simulink library "hcu_lib"  (Simulink 8.6)
settings: Solver=ode45  SolverMode=SingleTasking  StartTime=0.0  StopTime=10.0  RelTol=1e-3
PreLoadFcn:
  | if exist('tl_preloadfcn','file'), tl_preloadfcn(gcs,100); end
PostLoadFcn:
  | if exist('tl_postloadfcn','file'), tl_postloadfcn(gcs,100); end
undefined symbols (not defined in the file or in its folder): C_TICK_TIME_S, DEG2RAD, EPSILON, FALSE, RAD2DEG, TRUE
undefined symbols (not defined in the file): UNDEFINED_VALUE
libraries: hcu_lib x19, simulink x4
(part 1 of 3)
settings Model: TLRevision=100  Creator=gpf  LastModifiedBy=14069  ExtModeAutoUpdateStatusClock=off

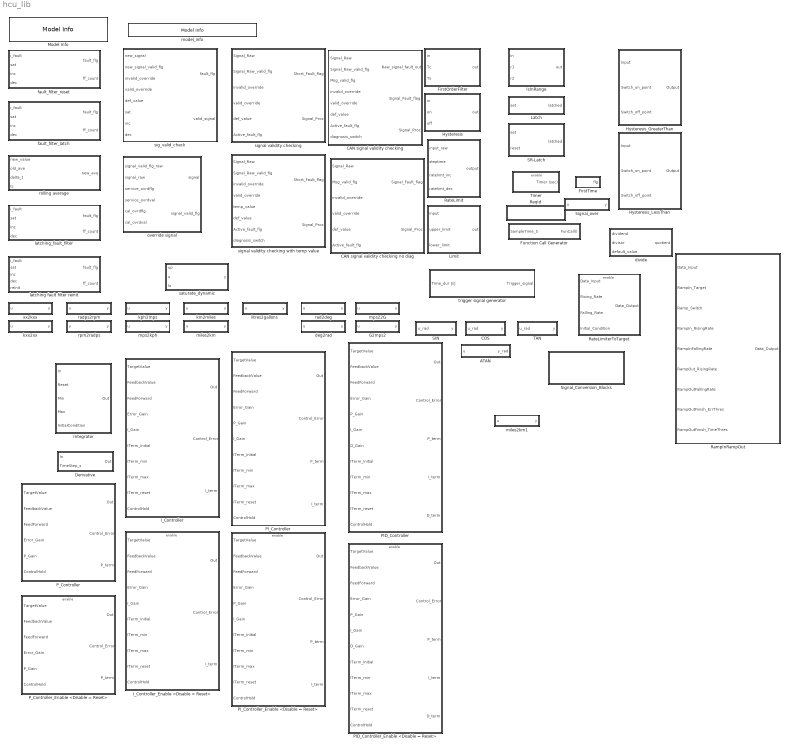
== system hcu_lib ==
  ATAN : Subsystem  TreatAsAtomicUnit=on  RTWFcnName=atan_lib  RTWFileName=HCU_LIB  mask(Inverse Trigonometric Function (ArcTangent)){}
      mask help:
      | Calculate aTan of the Input Signal.
      | The unit of output signal is rad.
      | If input signal is greater than 1000, it would be regard as PI rad.
      | If input signal is less than -1000, it would be regarded as -PI rad.
      | The output is bounded between -PI rad to PI rad.
      settings: RTWFcnNameOpts=User specified  RTWFileNameOpts=User specified
      mask Display:
      | disp('ATAN(X)' , 'texmode', 'on');
      | port_label('output',1,'Y_rad');
      | port_label('input',1,'X')
  CAN signal validity checking : Subsystem  TreatAsAtomicUnit=on  RTWFcnName=can_sig_valid_check  RTWFileName=HCU_LIB
      settings: RTWFcnNameOpts=User specified  RTWFileNameOpts=User specified
  CAN signal validity checking no diag : Subsystem  TreatAsAtomicUnit=on  RTWFcnName=can_sig_valid_check_no_diag  RTWFileName=HCU_LIB
      settings: RTWFcnNameOpts=User specified  RTWFileNameOpts=User specified
  COS : Subsystem  TreatAsAtomicUnit=on  RTWFcnName=cos_lib  RTWFileName=HCU_LIB  mask(Trigonometric Function (Cosine)){}
      mask help:
      | Calculate Cos of the Input Signal.
      | The unit of input signal is rad.
      settings: RTWFcnNameOpts=User specified  RTWFileNameOpts=User specified
      mask Display:
      | disp('       COS(X)' , 'texmode', 'on');
      | port_label('output',1,'Y');
      | port_label('input',1,'X_rad')
  Derivative : Subsystem  TreatAsAtomicUnit=on  RTWFcnName=derivative_lib  RTWFileName=HCU_LIB
      settings: RTWFcnNameOpts=User specified  RTWFileNameOpts=User specified
      mask Display: disp('Derivative')
  FirstOrderFilter : Subsystem  TreatAsAtomicUnit=on  RTWFcnName=firstorderfilter_lib  RTWFileName=HCU_LIB
      settings: RTWFcnNameOpts=User specified  RTWFileNameOpts=User specified
  FirstTime : Subsystem  TreatAsAtomicUnit=on  RTWFcnName=firsttime_lib  RTWFileName=HCU_LIB  mask(First Time True){}
      mask help: The output is TRUE if first time executing the block.
      settings: RTWFcnNameOpts=User specified  RTWFileNameOpts=User specified
  Function Call Generator : Stateflow chart  TreatAsAtomicUnit=on
  G2mps2 : Subsystem  TreatAsAtomicUnit=on  RTWFcnName=G2mps2_lib  RTWFileName=HCU_LIB  mask(Conversion){}
      mask help: Convert G to Meter per second^2.
      settings: RTWFcnNameOpts=User specified  RTWFileNameOpts=User specified
      mask Display: disp('G \rightarrow m/s2', 'texmode', 'on')
  Hysteresis : Subsystem  TreatAsAtomicUnit=on  RTWFcnName=hysteresis_lib  RTWFileName=HCU_LIB
      settings: RTWFcnNameOpts=User specified  RTWFileNameOpts=User specified
  Hysteresis_GreaterThan : Subsystem  TreatAsAtomicUnit=on  RTWFcnName=hysteresisgreaterthan_lib  RTWFileName=HCU_LIB
      settings: RTWFcnNameOpts=User specified  RTWFileNameOpts=User specified
  Hysteresis_LessThan : Subsystem  TreatAsAtomicUnit=on  RTWFcnName=hysteresislessthan_lib  RTWFileName=HCU_LIB
      settings: RTWFcnNameOpts=User specified  RTWFileNameOpts=User specified
  I_Controller : Subsystem  TreatAsAtomicUnit=on  RTWFcnName=icontroller_lib  RTWFileName=HCU_LIB
      settings: RTWFcnNameOpts=User specified  RTWFileNameOpts=User specified
      mask Display: disp('I Controller')
  I_Controller_Enable <Disable = Reset> : Subsystem  TreatAsAtomicUnit=on  RTWFcnName=icontrollerenable_lib  RTWFileName=HCU_LIB
      settings: RTWFcnNameOpts=User specified  RTWFileNameOpts=User specified
      mask Display: disp('I Controller\nwith Enable')
  Integrator : Subsystem  TreatAsAtomicUnit=on  RTWFcnName=integrator_lib  RTWFileName=HCU_LIB
      settings: RTWFcnNameOpts=User specified  RTWFileNameOpts=User specified
      mask Display: disp('Integrator')
  IsInRange : Subsystem  TreatAsAtomicUnit=on  RTWFcnName=isinrange_lib  RTWFileName=HCU_LIB
      settings: RTWFcnNameOpts=User specified  RTWFileNameOpts=User specified
  Latch : Subsystem  TreatAsAtomicUnit=on  RTWFcnName=latch_lib  RTWFileName=HCU_LIB
      settings: RTWFcnNameOpts=User specified  RTWFileNameOpts=User specified
  Limit : Subsystem  TreatAsAtomicUnit=on  RTWFcnName=limit_lib  RTWFileName=HCU_LIB
      settings: RTWFcnNameOpts=User specified  RTWFileNameOpts=User specified
  Model Info : simulink/Model-Wide Utilities/Model Info  BlockCM=None  Frame=on  DisplayStringWithTags=|  HorizontalTextAlignment=Left  LeftAlignmentValue=0.02  SourceBlockDiagram=hcu_lib  TagMaxNumber=20
      | Model Version        : %<ModelVersion>
      | Creator                   : %<Creator>
      | Last Modified by    : %<LastModifiedBy>
  PID_Controller : Subsystem  TreatAsAtomicUnit=on  RTWFcnName=pidcontroller_lib  RTWFileName=HCU_LIB
      settings: RTWFcnNameOpts=User specified  RTWFileNameOpts=User specified
      mask Display: disp('PID Controller')
  PID_Controller_Enable <Disable = Reset> : Subsystem  TreatAsAtomicUnit=on  RTWFcnName=pidcontrollerenable_lib  RTWFileName=HCU_LIB
      settings: RTWFcnNameOpts=User specified  RTWFileNameOpts=User specified
      mask Display: disp('PID Controller\nwith Enable')
  PI_Controller : Subsystem  TreatAsAtomicUnit=on  RTWFcnName=picontroller_lib  RTWFileName=HCU_LIB
      settings: RTWFcnNameOpts=User specified  RTWFileNameOpts=User specified
      mask Display: disp('PI Controller')
  PI_Controller_Enable <Disable = Reset> : Subsystem  TreatAsAtomicUnit=on  RTWFcnName=picontrollerenable_lib  RTWFileName=HCU_LIB
      settings: RTWFcnNameOpts=User specified  RTWFileNameOpts=User specified
      mask Display: disp('PI Controller\nwith Enable')
  P_Controller : Subsystem  TreatAsAtomicUnit=on  RTWFcnName=pcontroller_lib  RTWFileName=HCU_LIB
      settings: RTWFcnNameOpts=User specified  RTWFileNameOpts=User specified
      mask Display: disp('P Controller')
  P_Controller_Enable <Disable = Reset> : Subsystem  TreatAsAtomicUnit=on  RTWFcnName=pcontrollerenable_lib  RTWFileName=HCU_LIB
      settings: RTWFcnNameOpts=User specified  RTWFileNameOpts=User specified
      mask Display: disp('P Controller\nwith Enable')
  RampInRampOut : Subsystem  TreatAsAtomicUnit=on  RTWFcnName=rampinrampout_lib  RTWFileName=HCU_LIB
      settings: RTWFcnNameOpts=User specified  RTWFileNameOpts=User specified
  RateLimit : Subsystem  TreatAsAtomicUnit=on  RTWFcnName=ratelimit_lib  RTWFileName=HCU_LIB
      settings: RTWFcnNameOpts=User specified  RTWFileNameOpts=User specified
  RateLimiterToTarget : Subsystem  RTWFcnName=ratelimitertotarget_lib  RTWFileName=HCU_LIB
      settings: RTWFcnNameOpts=User specified  RTWFileNameOpts=User specified
  ReqId : Subsystem  mask(ReqId){req_str=HCU_000}
      mask prompts: req_str "Requirement:"
      mask help: Requirement Id
      mask Display: disp(sprintf('ReqId: %s',req_str));
  SIN : Subsystem  TreatAsAtomicUnit=on  RTWFcnName=sin_lib  RTWFileName=HCU_LIB  mask(Trigonometric Function (Sine)){}
      mask help:
      | Calculate Sin of the Input Signal.
      | The unit of input signal is rad.
      settings: RTWFcnNameOpts=User specified  RTWFileNameOpts=User specified
      mask Display:
      | disp('      SIN(X)' , 'texmode', 'on');
      | port_label('output',1,'Y');
      | port_label('input',1,'X_rad')
  SR-Latch : Subsystem  TreatAsAtomicUnit=on  RTWFcnName=srlatch_lib  RTWFileName=HCU_LIB
      settings: RTWFcnNameOpts=User specified  RTWFileNameOpts=User specified
  Signal_Conversion_Blocks : Subsystem
  Signal_over : Subsystem  mask(Override){parent_name=Signal, cal=0}
      mask prompts: parent_name "Name"; cal "Set Value"
      mask help: Override signal
      mask Callback parent_name: set_param(gcb, 'name', [get_param(gcb, 'parent_name') '_over']);
      mask Display: disp('Override');
  TAN : Subsystem  TreatAsAtomicUnit=on  RTWFcnName=tan_lib  RTWFileName=HCU_LIB  mask(Trigonometric Function (Tangent)){}
      mask help:
      | Calculate Tan of the Input Signal.
      | The unit of input signal is rad.
      settings: RTWFcnNameOpts=User specified  RTWFileNameOpts=User specified
      mask Display:
      | disp('      TAN(X)' , 'texmode', 'on');
      | port_label('output',1,'Y');
      | port_label('input',1,'X_rad')
  Timer : Subsystem  TreatAsAtomicUnit=on  RTWFcnName=timer_lib  RTWFileName=HCU_LIB
      settings: RTWFcnNameOpts=User specified  RTWFileNameOpts=User specified
  deg2rad : Subsystem  TreatAsAtomicUnit=on  RTWFcnName=deg2rad_lib  RTWFileName=HCU_LIB  mask(Conversion){}
      mask help: Convert degs to rads.
      settings: RTWFcnNameOpts=User specified  RTWFileNameOpts=User specified
      mask Display: disp('deg \rightarrow rad', 'texmode', 'on')
  divide : Subsystem  TreatAsAtomicUnit=on  RTWFcnName=divide_lib  RTWFileName=HCU_LIB  mask(divide){}
      mask help: Performs a division operation. If the divisor is found to be between -0.00001 and +0.00001 then a failsafe value is passed to the output.
      settings: RTWFcnNameOpts=User specified  RTWFileNameOpts=User specified
      mask Display: disp('Divide');
  fault_filter_latch : Subsystem  TreatAsAtomicUnit=on  RTWFcnName=ff_latch  RTWFileName=HCU_LIB
      settings: RTWFcnNameOpts=Use subsystem name  RTWFileNameOpts=User specified
  fault_filter_reset : Subsystem  TreatAsAtomicUnit=on  RTWFcnName=ff_reset  RTWFileName=HCU_LIB
      settings: RTWFcnNameOpts=User specified  RTWFileNameOpts=User specified
  km2miles : Subsystem  TreatAsAtomicUnit=on  RTWFcnName=km2miles_lib  RTWFileName=HCU_LIB  mask(Conversion){}
      mask help: Convert kilometers to miles.
      settings: RTWFcnNameOpts=User specified  RTWFileNameOpts=User specified
      mask Display: disp('km \rightarrow mile', 'texmode', 'on')
  kph2mps : Subsystem  TreatAsAtomicUnit=on  RTWFcnName=kph2mps_lib  RTWFileName=HCU_LIB  mask(Conversion){}
      mask help: Convert Kilometers per hour to Meters per second
      settings: RTWFcnNameOpts=User specified  RTWFileNameOpts=User specified
      mask Display: disp('km/h \rightarrow m/s', 'texmode', 'on')
  kxx2xx : Subsystem  TreatAsAtomicUnit=on  RTWFcnName=kxx2xx_lib  RTWFileName=HCU_LIB  mask(Conversion){}
      mask help: Multiply by 1000.
      settings: RTWFcnNameOpts=User specified  RTWFileNameOpts=User specified
      mask Display: disp('kiloxx \rightarrow xx', 'texmode', 'on')
  latching fault filter reinit : Subsystem  TreatAsAtomicUnit=on  RTWFcnName=ff_latching  RTWFileName=HCU_LIB  mask(Latching Fault Filter){}
      mask help: Fault filter block - Latches the fault output flag to TRUE if the input flag is repeatedly set True.
      settings: RTWFcnNameOpts=User specified  RTWFileNameOpts=User specified
      mask Display: disp('Latching\nFault Filter')
  latching_fault_filter : Subsystem  TreatAsAtomicUnit=on  RTWFcnName=ff_latching  RTWFileName=HCU_LIB  mask(Latching Fault Filter){}
      mask help: Fault filter block - Latches the fault output flag to TRUE if the input flag is repeatedly set True.
      settings: RTWFcnNameOpts=User specified  RTWFileNameOpts=User specified
      mask Display: disp('Latching\nFault Filter')
  litres2gallons : Subsystem  TreatAsAtomicUnit=on  RTWFcnName=liters2gallons_lib  RTWFileName=HCU_LIB  mask(Conversion){UK=off}
      mask prompts: UK "UK Gallon"
      mask help: Convert litres to gallons.
      settings: RTWFcnNameOpts=User specified  RTWFileNameOpts=User specified
      mask Display: disp('litre \rightarrow gallon', 'texmode', 'on')
  miles2km : Subsystem  TreatAsAtomicUnit=on  RTWFcnName=miles2km_lib  RTWFileName=HCU_LIB  mask(Conversion){}
      mask help: Convert kilometers to miles.
      settings: RTWFcnNameOpts=User specified  RTWFileNameOpts=User specified
      mask Display: disp('mile \rightarrow km', 'texmode', 'on')
  miles2km1 : Subsystem  mask(Conversion){}
      mask help: Convert degs to rads.
      mask Display: disp('deg \rightarrow rad', 'texmode', 'on')
  model_info : simulink/Model-Wide Utilities/Model Info  BlockCM=None  Frame=on  DisplayStringWithTags=$Id: hcu_lib.mdl 2 2019-09-19 09:28:50Z JuneXmas $  HorizontalTextAlignment=Center  LeftAlignmentValue=0.5  SourceBlockDiagram=hcu_lib  TagMaxNumber=20
  mps22G : Subsystem  TreatAsAtomicUnit=on  RTWFcnName=mps22G_lib  RTWFileName=HCU_LIB  mask(Conversion){}
      mask help: Convert Meter per second^2 to G.
      settings: RTWFcnNameOpts=User specified  RTWFileNameOpts=User specified
      mask Display: disp('m/s2 \rightarrow G', 'texmode', 'on')
  mps2kph : Subsystem  TreatAsAtomicUnit=on  RTWFcnName=mps2kph_lib  RTWFileName=HCU_LIB  mask(Conversion){}
      mask help: Convert Meters per second to Kilometers per hour
      settings: RTWFcnNameOpts=User specified  RTWFileNameOpts=User specified
      mask Display: disp('m/s \rightarrow km/h', 'texmode', 'on')
  override signal : Subsystem  RTWFcnName=srvc_ovrd  RTWFileName=HCU_LIB
      settings: RTWSystemCode=Inline  RTWFcnNameOpts=User specified  RTWFileNameOpts=User specified
  rad2deg : Subsystem  TreatAsAtomicUnit=on  RTWFcnName=rad2deg_lib  RTWFileName=HCU_LIB  mask(Conversion){}
      mask help: Convert rads to degs.
      settings: RTWFcnNameOpts=User specified  RTWFileNameOpts=User specified
      mask Display: disp('rad \rightarrow deg', 'texmode', 'on')
  radps2rpm : Subsystem  TreatAsAtomicUnit=on  RTWFcnName=radps2rpm_lib  RTWFileName=HCU_LIB
      mask help: Converst radians per second to revolutions per minute.
      settings: RTWFcnNameOpts=User specified  RTWFileNameOpts=User specified
      mask Display: disp('rad/s \rightarrow rpm', 'texmode', 'on')
  rolling average : Subsystem  TreatAsAtomicUnit=on  RTWFcnName=rolav_tc  RTWFileName=HCU_LIB  mask(Rolling Average){}
      mask help:
      | Rolling Average - Time Constant.  This filter block is the first order approximation using a time constant.  Inputs include the time constant (entered through this dialogue), old_ave which is the previous average value, new_value which is the new filter to filter toward.
      |
      | The sample_interval which is elapsed time over which to perform the filter equation is computed internally - THIS BLOCK MUST BE CALLED EACH PASS to work as expected.
      settings: RTWFcnNameOpts=User specified  RTWFileNameOpts=User specified
      mask Display: disp('Rolling Average - TC')
  rpm2radps : Subsystem  TreatAsAtomicUnit=on  RTWFcnName=rpm2radps_lib  RTWFileName=HCU_LIB
      mask help: Converts revolutions per minute to radians per second.
      settings: RTWFcnNameOpts=User specified  RTWFileNameOpts=User specified
      mask Display: disp('rpm \rightarrow rad/s', 'texmode', 'on')
  saturate_dynamic : Subsystem  TreatAsAtomicUnit=on  RTWFcnName=saturatedynamic_lib  RTWFileName=HCU_LIB  mask(saturate_dynamic){}
      mask help: Limit input signal in dynamic upper and lower limits
      settings: RTWFcnNameOpts=User specified  RTWFileNameOpts=User specified
      mask Display: disp('Saturate_Dynamic');
  sig_valid_check : Subsystem  TreatAsAtomicUnit=on  RTWFcnName=sig_valid_check  RTWFileName=HCU_LIB
      settings: RTWFcnNameOpts=User specified  RTWFileNameOpts=User specified
  signal validity checking : Subsystem  TreatAsAtomicUnit=on  RTWFcnName=sig_valid_check  RTWFileName=HCU_LIB
      settings: RTWFcnNameOpts=User specified  RTWFileNameOpts=User specified
  signal validity checking with temp value : Subsystem  TreatAsAtomicUnit=on  RTWFcnName=sig_valid_check_with_temp_value  RTWFileName=HCU_LIB
      settings: RTWFcnNameOpts=User specified  RTWFileNameOpts=User specified
  trigger signal generator : Subsystem  TreatAsAtomicUnit=on
  xx2kxx : Subsystem  TreatAsAtomicUnit=on  RTWFcnName=xx2kxx_lib  RTWFileName=HCU_LIB  mask(Conversion){}
      mask help: Divides by 1000.
      settings: RTWFcnNameOpts=User specified  RTWFileNameOpts=User specified
      mask Display: disp('xx \rightarrow kiloxx', 'texmode', 'on')

== system hcu_lib/ATAN ==
  u : Inport
  ATAN_Function_NEG : Lookup_n-D  NumberOfTableDimensions=1  BreakpointsForDimension1="[-1000\t-11.4300523\t-5.67128182\t-3.732050808\t-1.732050808\t-1\t-0.577350269\t-0.267949192\t-0.176326981\t-0.087488664\t0]"  Table="[-90\t-85\t-80\t-75\t-60\t-45\t-30\t-15\t-10\t-5\t0]"  ExtrapMethod=Clip  UseLastTableValue=on  InternalRulePriority=Speed  RndMeth=Simplest  InputSameDT=on
  ATAN_Function_POS : Lookup_n-D  NumberOfTableDimensions=1  BreakpointsForDimension1="[0\t0.087488664\t0.176326981\t0.267949192\t0.577350269\t1\t1.732050808\t3.732050808\t5.67128182\t11.4300523\t1000]"  Table="[0\t5\t10\t15\t30\t45\t60\t75\t80\t85\t90]"  ExtrapMethod=Clip  UseLastTableValue=on  InternalRulePriority=Speed  RndMeth=Simplest  InputSameDT=on
  Compare To Zero : simulink/Logic and Bit Operations/Compare To Zero  relop=>=  OutDataTypeStr=boolean
  Saturation : Saturate  UpperLimit=1000  LowerLimit=0
  Saturation1 : Saturate  UpperLimit=0  LowerLimit=-1000
  Switch : Switch  Criteria=u2 ~= 0
  deg2rad : hcu_lib/deg2rad
  y_rad : Outport
  wires:
  ATAN_Function_POS/1 -> Switch/1
  Saturation/1 -> ATAN_Function_POS/1
  Saturation1/1 -> ATAN_Function_NEG/1
  u/1 -> Saturation/1, Compare To Zero/1, Saturation1/1
  ATAN_Function_NEG/1 -> Switch/3
  Compare To Zero/1 -> Switch/2
  Switch/1 -> deg2rad/1
  deg2rad/1 -> y_rad/1

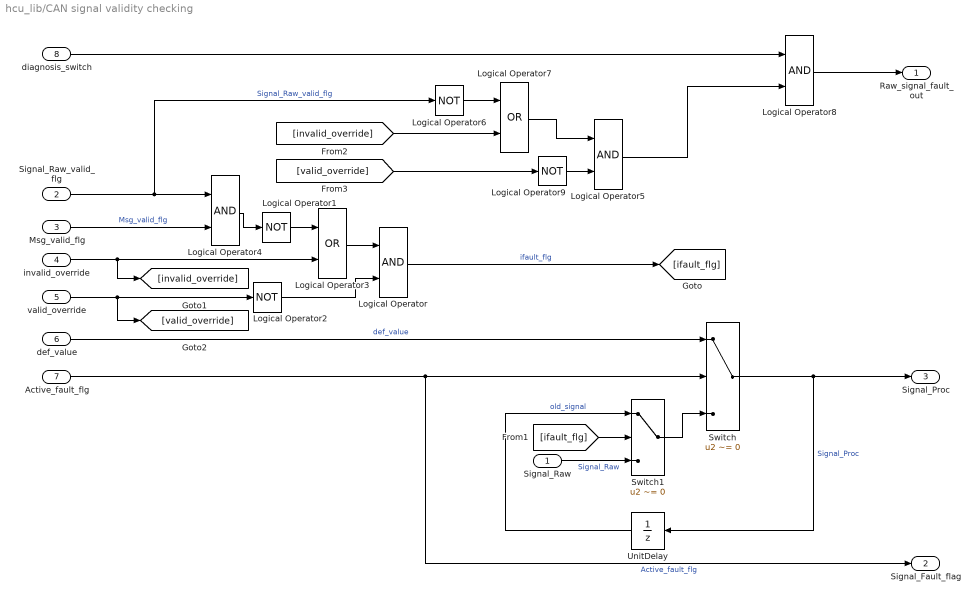
== system hcu_lib/CAN signal validity checking ==
  Signal_Raw : Inport
  Signal_Raw_valid_flg : Inport  Port=2
  Msg_valid_flg : Inport  Port=3
  invalid_override : Inport  Port=4
  valid_override : Inport  Port=5
  def_value : Inport  Port=6
  Active_fault_flg : Inport  Port=7
  diagnosis_switch : Inport  Port=8
  Logical Operator{,4..5,8} (4 alike) : Logic  Tag=struct('inputs','2','comment',struct('text','','placement',1),'logdata',struct('maxnumvals',inf,'plotchannels',[],'stepsize',0,'downsampling',1,'loggingmode',3,'channels',1),'operator','OR','output',struct('class','default','type','Bool8','description','','address','','unit','','name','$S_$B'),'date',731430.467498704)
  Logical Operator{1..2,6,9} (4 alike) : Logic  Tag=struct('inputs','1','comment',struct('text','','placement',1),'logdata',struct('maxnumvals',inf,'plotchannels',[],'stepsize',0,'downsampling',1,'loggingmode',3,'channels',1),'operator','NOT','output',struct('class','default','type','Bool8','description','','address','','unit','','name','$S_$B'),'date',731430.46749816)  Operator=NOT  Inputs=1
  Logical Operator3 : Logic  Tag=struct('inputs','2','comment',struct('text','','placement',1),'logdata',struct('maxnumvals',inf,'plotchannels',[],'stepsize',0,'downsampling',1,'loggingmode',3,'channels',1),'operator','OR','output',struct('class','default','type','Bool8','description','','address','','unit','','name','$S_$B'),'date',731430.467498704)  Operator=OR
  Logical Operator7 : Logic  Tag=struct('inputs','2','comment',struct('text','','placement',1),'logdata',struct('maxnumvals',inf,'plotchannels',[],'stepsize',0,'downsampling',1,'loggingmode',3,'channels',1),'operator','OR','output',struct('class','default','type','Bool8','description','','address','','unit','','name','$S_$B'),'date',731430.467498704)  Operator=OR
  Switch : Switch  Criteria=u2 ~= 0
  Switch1 : Switch  Criteria=u2 ~= 0
  UnitDelay : UnitDelay  Tag=struct('comment',struct('text','','placement',1),'logdata',struct('maxnumvals',inf,'plotchannels',[],'stepsize',0,'downsampling',1,'loggingmode',3,'channels',1),'output',struct('width',1,'name','$S_$B','unit','','type','Int32Bin15','offset',0,'max',32767,'min',-32768,'freeze',1,'lsb',2^-16,'arb',0,'class','default','address','','description','','autoscalingmode',1,'lowerheadroom',1,'upperheadroom',1,'headroomunit','bit','checkmin',0,'checkmax',0,'show',0,'initial','0'),'state',0,'dt','-1','date',731401.644401968)  SampleTime=-1
  Raw_signal_fault_out : Outport
  Signal_Fault_flag : Outport  Port=2
  Signal_Proc : Outport  Port=3
  wires:
  Logical Operator6/1 -> Logical Operator7/1
  Logical Operator9/1 -> Logical Operator5/2
  diagnosis_switch/1 -> Logical Operator8/1
  Logical Operator8/1 -> Raw_signal_fault_out/1
  Logical Operator5/1 -> Logical Operator8/2
  Logical Operator7/1 -> Logical Operator5/1
  [invalid_override] -> Logical Operator7/2
  [valid_override] -> Logical Operator9/1
  Logical Operator4/1 -> Logical Operator1/1
  Msg_valid_flg/1 -> Logical Operator4/2  "Msg_valid_flg"
  Switch/1 -> Signal_Proc/1, UnitDelay/1  "Signal_Proc"
  def_value/1 -> Switch/1  "def_value"
  Logical Operator1/1 -> Logical Operator3/1
  Signal_Raw_valid_flg/1 -> Logical Operator6/1, Logical Operator4/1  "Signal_Raw_valid_flg"
  invalid_override/1 -> [invalid_override], Logical Operator3/2
  Active_fault_flg/1 -> Signal_Fault_flag/1, Switch/2  "Active_fault_flg"
  UnitDelay/1 -> Switch1/1  "old_signal"
  Switch1/1 -> Switch/3
  Signal_Raw/1 -> Switch1/3  "Signal_Raw"
  Logical Operator/1 -> [ifault_flg]  "ifault_flg"
  [ifault_flg] -> Switch1/2
  valid_override/1 -> [valid_override], Logical Operator2/1
  Logical Operator3/1 -> Logical Operator/1
  Logical Operator2/1 -> Logical Operator/2

== system hcu_lib/CAN signal validity checking no diag ==
  Signal_Raw : Inport
  Msg_valid_flg : Inport  Port=2
  invalid_override : Inport  Port=3
  valid_override : Inport  Port=4
  def_value : Inport  Port=5
  Active_fault_flg : Inport  Port=6
  Logical Operator : Logic  Tag=struct('inputs','2','comment',struct('text','','placement',1),'logdata',struct('maxnumvals',inf,'plotchannels',[],'stepsize',0,'downsampling',1,'loggingmode',3,'channels',1),'operator','OR','output',struct('class','default','type','Bool8','description','','address','','unit','','name','$S_$B'),'date',731430.467498704)
  Logical Operator1 : Logic  Tag=struct('inputs','1','comment',struct('text','','placement',1),'logdata',struct('maxnumvals',inf,'plotchannels',[],'stepsize',0,'downsampling',1,'loggingmode',3,'channels',1),'operator','NOT','output',struct('class','default','type','Bool8','description','','address','','unit','','name','$S_$B'),'date',731430.46749816)  Operator=NOT  Inputs=1
  Logical Operator2 : Logic  Tag=struct('inputs','1','comment',struct('text','','placement',1),'logdata',struct('maxnumvals',inf,'plotchannels',[],'stepsize',0,'downsampling',1,'loggingmode',3,'channels',1),'operator','NOT','output',struct('class','default','type','Bool8','description','','address','','unit','','name','$S_$B'),'date',731430.46749816)  Operator=NOT  Inputs=1
  Logical Operator3 : Logic  Tag=struct('inputs','2','comment',struct('text','','placement',1),'logdata',struct('maxnumvals',inf,'plotchannels',[],'stepsize',0,'downsampling',1,'loggingmode',3,'channels',1),'operator','OR','output',struct('class','default','type','Bool8','description','','address','','unit','','name','$S_$B'),'date',731430.467498704)  Operator=OR
  Switch : Switch  Criteria=u2 ~= 0
  Switch1 : Switch  Criteria=u2 ~= 0
  UnitDelay : UnitDelay  Tag=struct('comment',struct('text','','placement',1),'logdata',struct('maxnumvals',inf,'plotchannels',[],'stepsize',0,'downsampling',1,'loggingmode',3,'channels',1),'output',struct('width',1,'name','$S_$B','unit','','type','Int32Bin15','offset',0,'max',32767,'min',-32768,'freeze',1,'lsb',2^-16,'arb',0,'class','default','address','','description','','autoscalingmode',1,'lowerheadroom',1,'upperheadroom',1,'headroomunit','bit','checkmin',0,'checkmax',0,'show',0,'initial','0'),'state',0,'dt','-1','date',731401.644401968)  SampleTime=-1
  Signal_Fault_flag : Outport
  Signal_Proc : Outport  Port=2
  wires:
  Msg_valid_flg/1 -> Logical Operator1/1  "Msg_valid_flg"
  Switch/1 -> Signal_Proc/1, UnitDelay/1  "Signal_Proc"
  def_value/1 -> Switch/1  "def_value"
  Logical Operator1/1 -> Logical Operator3/1
  invalid_override/1 -> Logical Operator3/2
  Active_fault_flg/1 -> Signal_Fault_flag/1, Switch/2  "Active_fault_flg"
  UnitDelay/1 -> Switch1/1  "old_signal"
  Switch1/1 -> Switch/3
  Signal_Raw/1 -> Switch1/3  "Signal_Raw"
  Logical Operator/1 -> [ifault_flg]  "ifault_flg"
  [ifault_flg] -> Switch1/2
  valid_override/1 -> Logical Operator2/1
  Logical Operator3/1 -> Logical Operator/1
  Logical Operator2/1 -> Logical Operator/2

== system hcu_lib/COS ==
  u_rad : Inport
  COS_Function : Lookup_n-D  NumberOfTableDimensions=1  BreakpointsForDimension1="[0\t5\t10\t15\t30\t45\t60\t75\t80\t85\t90\t95\t100\t105\t120\t135\t150\t165\t170\t175\t180\t185\t190\t195\t210\t225\t240\t255\t260\t265\t270\t275\t280\t285\t300\t315\t330\t345\t350\t355\t360]"  Table="[1\t0.996194698\t0.984807753\t0.965925826\t0.866025404\t0.707106781\t0.5\t0.258819045\t0.173648178\t0.087155743\t0\t-0.087155743\t-0.173648178\t-0.258819045\t-0.5\t-0.707106781\t-0.866025404\t-0.965925826\t-0.984807753\t-0.996194698\t-1\t-0.996194698\t-0.984807753\t-0.965925826\t-0.866025404\t-0.707106781\t-0.5\t-0.258819045\t-0.173648178\t-0.087155743\t0\t0.087155743\t0.173648178\t0.258819045\t0.5\t0.707106781\t0.866025404\t0.965925826\t0.984807753\t0.996194698\t1]"  ExtrapMethod=Clip  UseLastTableValue=on  InternalRulePriority=Speed  RndMeth=Simplest  InputSameDT=on
  Constant : Constant  Value=single(2*pi)
  Gain : Gain  Gain=2*pi
  Product : Product  Inputs=*/
  Rounding Function : Rounding
  Saturation : Saturate  UpperLimit=360  LowerLimit=0
  Subtract : Sum  Inputs=+-
  km2miles1 : Subsystem  mask(Conversion){}
      mask help: Convert rads to degs.
      mask Display: disp('rad \rightarrow deg', 'texmode', 'on')
  y : Outport
  wires:
  Subtract/1 -> km2miles1/1(u)
  Gain/1 -> Subtract/2
  Rounding Function/1 -> Gain/1
  Product/1 -> Rounding Function/1
  Constant/1 -> Product/2
  u_rad/1 -> Subtract/1, Product/1
  km2miles1/1(y) -> Saturation/1
  Saturation/1 -> COS_Function/1
  COS_Function/1 -> y/1

== system hcu_lib/Derivative ==
  In : Inport
  TimeStep_s : Inport  Port=2
  DeltaInput : Subsystem  TreatAsAtomicUnit=on
  Function Call Generator : Stateflow chart  TreatAsAtomicUnit=on
  Product1 : Product  Inputs=*/
  Out : Outport
  wires:
  TimeStep_s/1 -> Product1/2, Function Call Generator/1(SampleTime_S)
  Function Call Generator/1(FunCall()) -> DeltaInput/Trigger
  In/1 -> DeltaInput/1(In1)
  DeltaInput/1(Out1) -> Product1/1
  Product1/1 -> Out/1

== system hcu_lib/FirstOrderFilter ==
  in : Inport
  Tc : Inport  Port=2
  Ts : Inport  Port=3
  Add : Sum
  Add1 : Sum
  Add2 : Sum  Inputs=+-
  Constant : Constant  OutDataTypeStr=single
  Divide : Product  Inputs=*/
  Product : Product  RndMeth=Zero
  Product1 : Product  RndMeth=Zero
  Unit Delay : UnitDelay  SampleTime=-1
  out : Outport
  wires:
  Unit Delay/1 -> Product1/2
  Tc/1 -> Add1/1, Divide/1
  Ts/1 -> Add1/2
  Add1/1 -> Divide/2
  Constant/1 -> Add2/1
  Divide/1 -> Add2/2, Product1/1
  in/1 -> Product/1
  Add2/1 -> Product/2
  Product/1 -> Add/1
  Product1/1 -> Add/2
  Add/1 -> out/1, Unit Delay/1

== system hcu_lib/FirstTime ==
  FALSE : Constant  Value=FALSE
  Unit Delay : UnitDelay  InitialCondition=TRUE  SampleTime=-1
  flg : Outport
  wires:
  FALSE/1 -> Unit Delay/1
  Unit Delay/1 -> flg/1

== system hcu_lib/G2mps2 ==
  u : Inport
  Gain : Gain  Gain=9.81
  y : Outport
  wires:
  Gain/1 -> y/1  "y"
  u/1 -> Gain/1  "u"

== system hcu_lib/Hysteresis ==
  in : Inport
  on : Inport  Port=2
  off : Inport  Port=3
  Logical Operator1 : Logic  AllPortsSameDT=off  OutDataTypeStr=boolean
  Logical Operator2 : Logic  AllPortsSameDT=off  OutDataTypeStr=boolean
  Logical Operator3 : Logic  Operator=NOT  AllPortsSameDT=off  OutDataTypeStr=boolean
  RESET : Constant  Value=0  OutDataTypeStr=boolean
  Relational Operator1 : RelationalOperator  OutDataTypeStr=boolean
  Relational Operator2 : RelationalOperator  Operator=<  OutDataTypeStr=boolean
  SET : Constant  OutDataTypeStr=boolean
  Switch : Switch  Criteria=u2 ~= 0
  Switch1 : Switch  Criteria=u2 ~= 0
  Unit Delay : UnitDelay  SampleTime=-1
  out : Outport
  wires:
  in/1 -> Relational Operator1/1, Relational Operator2/1
  on/1 -> Relational Operator1/2
  off/1 -> Relational Operator2/2
  Relational Operator1/1 -> Logical Operator1/1
  Relational Operator2/1 -> Logical Operator2/1
  Logical Operator1/1 -> Switch/2
  SET/1 -> Switch/1
  Switch/1 -> Switch1/3
  Logical Operator2/1 -> Switch1/2
  RESET/1 -> Switch1/1
  Switch1/1 -> out/1, Unit Delay/1
  Unit Delay/1 -> Switch/3, Logical Operator3/1, Logical Operator2/2
  Logical Operator3/1 -> Logical Operator1/2

== system hcu_lib/Hysteresis_GreaterThan ==
  Input : Inport
  Switch_on_point : Inport  Port=2
  Switch_off_point : Inport  Port=3
  Logical Operator1 : Logic  AllPortsSameDT=off  OutDataTypeStr=boolean
  Logical Operator2 : Logic  Operator=NOT  AllPortsSameDT=off  OutDataTypeStr=boolean
  Logical Operator3 : Logic  Operator=OR  AllPortsSameDT=off  OutDataTypeStr=boolean
  Relational Operator : RelationalOperator  OutDataTypeStr=boolean
  Relational Operator1 : RelationalOperator  Operator=<=  OutDataTypeStr=boolean
  Unit Delay : UnitDelay  SampleTime=-1
  Output : Outport
  wires:
  Switch_on_point/1 -> Relational Operator/2
  Switch_off_point/1 -> Relational Operator1/2
  Logical Operator2/1 -> Logical Operator1/2
  Unit Delay/1 -> Logical Operator3/1
  Input/1 -> Relational Operator/1, Relational Operator1/1
  Relational Operator/1 -> Logical Operator3/2
  Logical Operator3/1 -> Logical Operator1/1
  Relational Operator1/1 -> Logical Operator2/1
  Logical Operator1/1 -> Output/1, Unit Delay/1

== system hcu_lib/Hysteresis_LessThan ==
  Input : Inport
  Switch_on_point : Inport  Port=2
  Switch_off_point : Inport  Port=3
  Logical Operator1 : Logic  AllPortsSameDT=off  OutDataTypeStr=boolean
  Logical Operator2 : Logic  Operator=NOT  AllPortsSameDT=off  OutDataTypeStr=boolean
  Logical Operator3 : Logic  Operator=OR  AllPortsSameDT=off  OutDataTypeStr=boolean
  Relational Operator : RelationalOperator  Operator=<=  OutDataTypeStr=boolean
  Relational Operator1 : RelationalOperator  OutDataTypeStr=boolean
  Unit Delay : UnitDelay  SampleTime=-1
  Output : Outport
  wires:
  Switch_on_point/1 -> Relational Operator/2
  Switch_off_point/1 -> Relational Operator1/2
  Logical Operator2/1 -> Logical Operator1/2
  Unit Delay/1 -> Logical Operator3/1
  Input/1 -> Relational Operator/1, Relational Operator1/1
  Relational Operator/1 -> Logical Operator3/2
  Logical Operator3/1 -> Logical Operator1/1
  Relational Operator1/1 -> Logical Operator2/1
  Logical Operator1/1 -> Output/1, Unit Delay/1

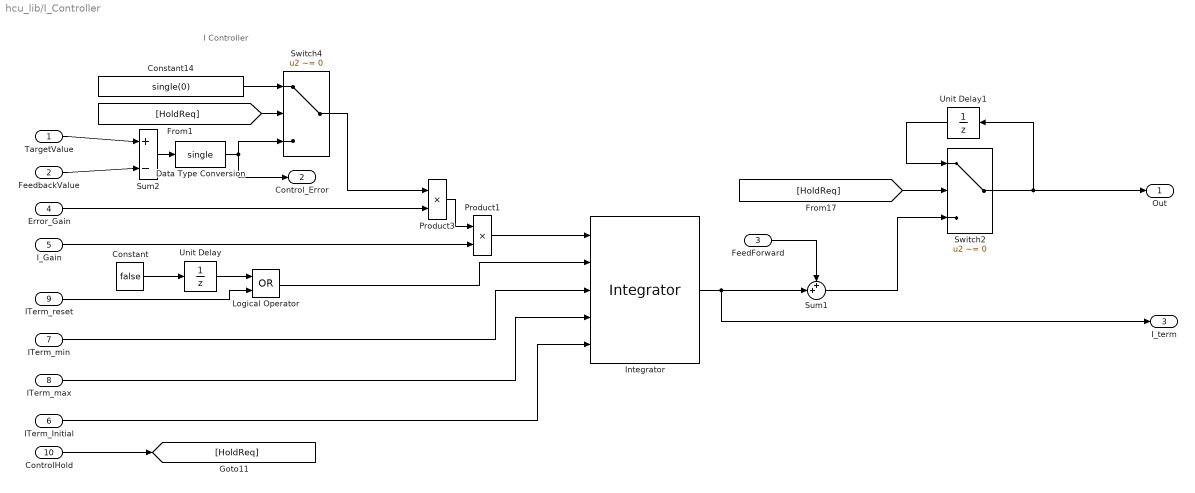
== system hcu_lib/I_Controller ==
  note: I Controller
  TargetValue : Inport
  FeedbackValue : Inport  Port=2
  FeedForward : Inport  Port=3
  Error_Gain : Inport  Port=4
  I_Gain : Inport  Port=5
  ITerm_Initial : Inport  Port=6
  ITerm_min : Inport  Port=7
  ITerm_max : Inport  Port=8
  ITerm_reset : Inport  Port=9
  ControlHold : Inport  Port=10
  Constant : Constant  Value=false  OutDataTypeStr=boolean
  Constant14 : Constant  Value=single(0)
  Data Type Conversion : DataTypeConversion  OutDataTypeStr=single  SaturateOnIntegerOverflow=on  RndMeth=Zero
  Integrator : hcu_lib/Integrator  SystemSampleTime=-1
  Logical Operator : Logic  Operator=OR  AllPortsSameDT=off  OutDataTypeStr=boolean
  Product1 : Product  InputSameDT=on  OutDataTypeStr=Inherit: Same as first input
  Product3 : Product  InputSameDT=on  OutDataTypeStr=Inherit: Same as first input
  Sum1 : Sum  Inputs=++|
  Sum2 : Sum  Inputs=+|-  SaturateOnIntegerOverflow=on  InputSameDT=on  OutDataTypeStr=Inherit: Same as first input
  Switch2 : Switch  Criteria=u2 ~= 0
  Switch4 : Switch  Criteria=u2 ~= 0
  Unit Delay : UnitDelay  InitialCondition=true  SampleTime=-1
  Unit Delay1 : UnitDelay  SampleTime=-1
  Out : Outport  OutputWhenDisabled=reset  InitialOutput=[0]
  Control_Error : Outport  Port=2  OutputWhenDisabled=reset  InitialOutput=[0]
  I_term : Outport  Port=3  OutputWhenDisabled=reset  InitialOutput=[0]
  wires:
  FeedbackValue/1 -> Sum2/2
  TargetValue/1 -> Sum2/1
  ITerm_max/1 -> Integrator/4
  ITerm_min/1 -> Integrator/3
  Error_Gain/1 -> Product3/2
  I_Gain/1 -> Product1/2
  Product1/1 -> Integrator/1
  Integrator/1 -> Sum1/2, I_term/1
  Product3/1 -> Product1/1
  Sum2/1 -> Data Type Conversion/1
  Logical Operator/1 -> Integrator/2
  ITerm_reset/1 -> Logical Operator/2
  Unit Delay/1 -> Logical Operator/1
  Constant/1 -> Unit Delay/1
  ControlHold/1 -> [HoldReq]
  [HoldReq] -> Switch2/2
  Switch2/1 -> Out/1, Unit Delay1/1
  Unit Delay1/1 -> Switch2/1
  Switch4/1 -> Product3/1
  Data Type Conversion/1 -> Control_Error/1, Switch4/3
  [HoldReq] -> Switch4/2
  Constant14/1 -> Switch4/1
  Sum1/1 -> Switch2/3
  FeedForward/1 -> Sum1/1
  ITerm_Initial/1 -> Integrator/5

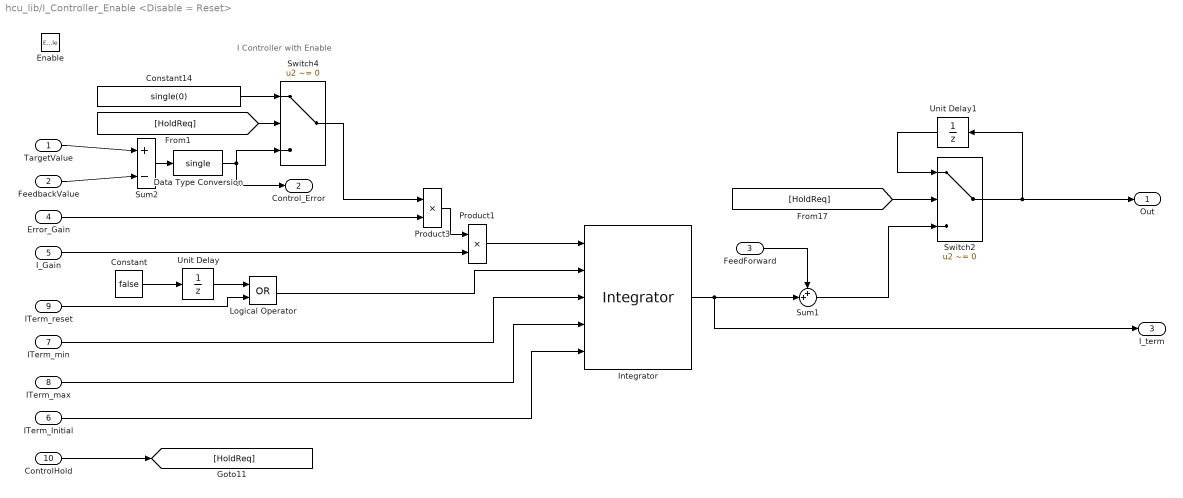
== system hcu_lib/I_Controller_Enable <Disable = Reset> ==
  note: I Controller with Enable
  TargetValue : Inport
  FeedbackValue : Inport  Port=2
  FeedForward : Inport  Port=3
  Error_Gain : Inport  Port=4
  I_Gain : Inport  Port=5
  ITerm_Initial : Inport  Port=6
  ITerm_min : Inport  Port=7
  ITerm_max : Inport  Port=8
  ITerm_reset : Inport  Port=9
  ControlHold : Inport  Port=10
  Enable : EnablePort  StatesWhenEnabling=reset
  Constant : Constant  Value=false  OutDataTypeStr=boolean
  Constant14 : Constant  Value=single(0)
  Data Type Conversion : DataTypeConversion  OutDataTypeStr=single  SaturateOnIntegerOverflow=on  RndMeth=Zero
  Integrator : hcu_lib/Integrator  SystemSampleTime=-1
  Logical Operator : Logic  Operator=OR  AllPortsSameDT=off  OutDataTypeStr=boolean
  Product1 : Product  InputSameDT=on  OutDataTypeStr=Inherit: Same as first input
  Product3 : Product  InputSameDT=on  OutDataTypeStr=Inherit: Same as first input
  Sum1 : Sum  Inputs=++|
  Sum2 : Sum  Inputs=+|-  SaturateOnIntegerOverflow=on  InputSameDT=on  OutDataTypeStr=Inherit: Same as first input
  Switch2 : Switch  Criteria=u2 ~= 0
  Switch4 : Switch  Criteria=u2 ~= 0
  Unit Delay : UnitDelay  InitialCondition=true  SampleTime=-1
  Unit Delay1 : UnitDelay  SampleTime=-1
  Out : Outport  OutputWhenDisabled=reset  InitialOutput=[0]
  Control_Error : Outport  Port=2  OutputWhenDisabled=reset  InitialOutput=[0]
  I_term : Outport  Port=3  OutputWhenDisabled=reset  InitialOutput=[0]
  wires:
  FeedForward/1 -> Sum1/1
  Sum1/1 -> Switch2/3
  Constant14/1 -> Switch4/1
  [HoldReq] -> Switch4/2
  Data Type Conversion/1 -> Switch4/3, Control_Error/1
  Switch4/1 -> Product3/1
  Unit Delay1/1 -> Switch2/1
  Switch2/1 -> Unit Delay1/1, Out/1
  [HoldReq] -> Switch2/2
  ControlHold/1 -> [HoldReq]
  Constant/1 -> Unit Delay/1
  Unit Delay/1 -> Logical Operator/1
  ITerm_reset/1 -> Logical Operator/2
  Logical Operator/1 -> Integrator/2
  Sum2/1 -> Data Type Conversion/1
  Product3/1 -> Product1/1
  Integrator/1 -> I_term/1, Sum1/2
  Product1/1 -> Integrator/1
  I_Gain/1 -> Product1/2
  Error_Gain/1 -> Product3/2
  ITerm_min/1 -> Integrator/3
  ITerm_max/1 -> Integrator/4
  TargetValue/1 -> Sum2/1
  FeedbackValue/1 -> Sum2/2
  ITerm_Initial/1 -> Integrator/5

== system hcu_lib/Integrator ==
  In : Inport
  Reset : Inport  Port=2
  Min : Inport  Port=3
  Max : Inport  Port=4
  InitialCondition : Inport  Port=5
  Constant : Constant  Value=C_TICK_TIME_S  OutDataTypeStr=single
  Data Type Conversion : DataTypeConversion  OutDataTypeStr=boolean  RndMeth=Zero
  Limit : hcu_lib/Limit  SystemSampleTime=-1
  Product : Product  SaturateOnIntegerOverflow=on  InputSameDT=on  OutDataTypeStr=Inherit: Same as first input
  Sum : Sum  Inputs=++|  SaturateOnIntegerOverflow=on  InputSameDT=on
  Switch1 : Switch  Criteria=u2 ~= 0  Threshold=1  ZeroCross=off  SaturateOnIntegerOverflow=on  InputSameDT=on
  Unit Delay : UnitDelay  SampleTime=-1
  Out : Outport
  wires:
  InitialCondition/1 -> Switch1/1
  Data Type Conversion/1 -> Switch1/2
  Reset/1 -> Data Type Conversion/1
  Unit Delay/1 -> Switch1/3
  Product/1 -> Sum/2
  In/1 -> Product/1
  Constant/1 -> Product/2
  Switch1/1 -> Sum/1, Out/1
  Sum/1 -> Limit/1
  Limit/1 -> Unit Delay/1
  Max/1 -> Limit/2
  Min/1 -> Limit/3

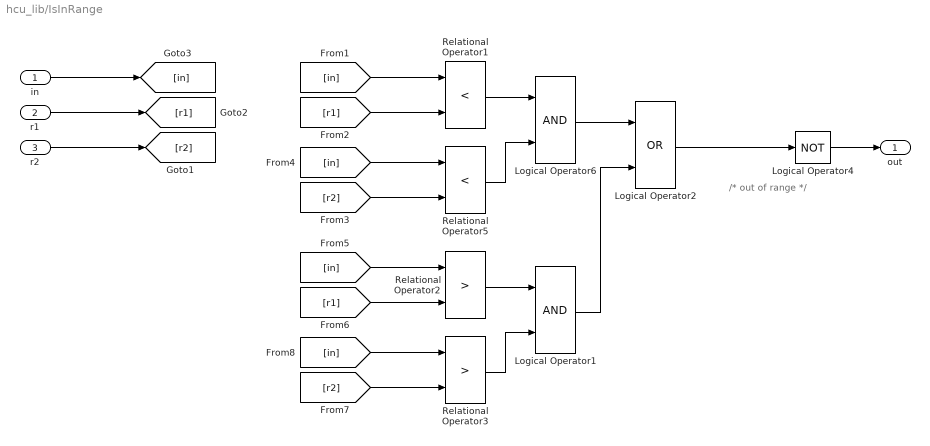
== system hcu_lib/IsInRange ==
  note: /* out of range */
  in : Inport
  r1 : Inport  Port=2
  r2 : Inport  Port=3
  Logical Operator1 : Logic  AllPortsSameDT=off  OutDataTypeStr=boolean
  Logical Operator2 : Logic  Operator=OR  AllPortsSameDT=off  OutDataTypeStr=boolean
  Logical Operator4 : Logic  Operator=NOT  AllPortsSameDT=off  OutDataTypeStr=boolean
  Logical Operator6 : Logic  AllPortsSameDT=off  OutDataTypeStr=boolean
  Relational Operator1 : RelationalOperator  Operator=<  OutDataTypeStr=boolean
  Relational Operator2 : RelationalOperator  Operator=>  OutDataTypeStr=boolean
  Relational Operator3 : RelationalOperator  Operator=>  OutDataTypeStr=boolean
  Relational Operator5 : RelationalOperator  Operator=<  OutDataTypeStr=boolean
  out : Outport
  wires:
  Relational Operator1/1 -> Logical Operator6/1
  Relational Operator5/1 -> Logical Operator6/2
  Logical Operator6/1 -> Logical Operator2/1
  in/1 -> [in]
  r1/1 -> [r1]
  r2/1 -> [r2]
  [in] -> Relational Operator1/1
  [r1] -> Relational Operator1/2
  [in] -> Relational Operator5/1
  [r2] -> Relational Operator5/2
  Relational Operator2/1 -> Logical Operator1/1
  Relational Operator3/1 -> Logical Operator1/2
  [in] -> Relational Operator2/1
  [r1] -> Relational Operator2/2
  [in] -> Relational Operator3/1
  [r2] -> Relational Operator3/2
  Logical Operator1/1 -> Logical Operator2/2
  Logical Operator2/1 -> Logical Operator4/1
  Logical Operator4/1 -> out/1

== system hcu_lib/Latch ==
  set : Inport
  Switch1 : Switch  Criteria=u2 ~= 0  Threshold=0.5
      settings: AttributesFormatString=<Criteria=%<Criteria>>
  Unit Delay : UnitDelay  SampleTime=-1
  latched : Outport
  wires:
  Unit Delay/1 -> Switch1/1, Switch1/2
  Switch1/1 -> Unit Delay/1, latched/1
  set/1 -> Switch1/3

== system hcu_lib/Limit ==
  input : Inport
  upper_limit : Inport  Port=2
  lower_limit : Inport  Port=3
  MinMax10 : MinMax  Function=max  Inputs=2
  MinMax5 : MinMax  Inputs=2
  out : Outport
  wires:
  lower_limit/1 -> MinMax10/2
  upper_limit/1 -> MinMax5/2
  MinMax10/1 -> out/1
  input/1 -> MinMax5/1
  MinMax5/1 -> MinMax10/1

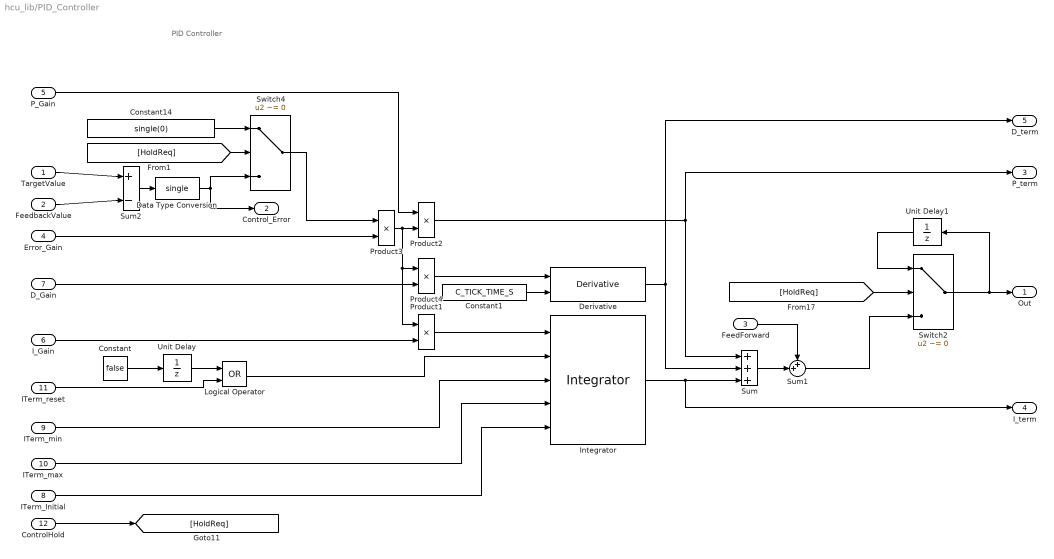
== system hcu_lib/PID_Controller ==
  note: PID Controller
  TargetValue : Inport
  FeedbackValue : Inport  Port=2
  FeedForward : Inport  Port=3
  Error_Gain : Inport  Port=4
  P_Gain : Inport  Port=5
  I_Gain : Inport  Port=6
  D_Gain : Inport  Port=7
  ITerm_Initial : Inport  Port=8
  ITerm_min : Inport  Port=9
  ITerm_max : Inport  Port=10
  ITerm_reset : Inport  Port=11
  ControlHold : Inport  Port=12
  Constant : Constant  Value=false  OutDataTypeStr=boolean
  Constant1 : Constant  Value=C_TICK_TIME_S  OutDataTypeStr=single
  Constant14 : Constant  Value=single(0)
  Data Type Conversion : DataTypeConversion  OutDataTypeStr=single  SaturateOnIntegerOverflow=on  RndMeth=Zero
  Derivative : hcu_lib/Derivative  SystemSampleTime=-1
  Integrator : hcu_lib/Integrator  SystemSampleTime=-1
  Logical Operator : Logic  Operator=OR  AllPortsSameDT=off  OutDataTypeStr=boolean
  Product{1..4} (4 alike) : Product  InputSameDT=on  OutDataTypeStr=Inherit: Same as first input
  Sum : Sum  Inputs=+++  SaturateOnIntegerOverflow=on  InputSameDT=on  OutDataTypeStr=Inherit: Same as first input
  Sum1 : Sum  Inputs=++|
  Sum2 : Sum  Inputs=+|-  SaturateOnIntegerOverflow=on  InputSameDT=on  OutDataTypeStr=Inherit: Same as first input
  Switch2 : Switch  Criteria=u2 ~= 0
  Switch4 : Switch  Criteria=u2 ~= 0
  Unit Delay : UnitDelay  InitialCondition=true  SampleTime=-1
  Unit Delay1 : UnitDelay  SampleTime=-1
  Out : Outport  OutputWhenDisabled=reset  InitialOutput=[0]
  Control_Error : Outport  Port=2  OutputWhenDisabled=reset  InitialOutput=[0]
  P_term : Outport  Port=3  OutputWhenDisabled=reset  InitialOutput=[0]
  I_term : Outport  Port=4  OutputWhenDisabled=reset  InitialOutput=[0]
  D_term : Outport  Port=5  OutputWhenDisabled=reset  InitialOutput=[0]
  wires:
  ITerm_Initial/1 -> Integrator/5
  FeedbackValue/1 -> Sum2/2
  TargetValue/1 -> Sum2/1
  ITerm_max/1 -> Integrator/4
  ITerm_min/1 -> Integrator/3
  Error_Gain/1 -> Product3/2
  P_Gain/1 -> Product2/1
  I_Gain/1 -> Product1/2
  Product1/1 -> Integrator/1
  Product2/1 -> P_term/1, Sum/1
  Integrator/1 -> Sum/3, I_term/1
  Sum/1 -> Sum1/2
  Product3/1 -> Product2/2, Product4/1, Product1/1
  Sum2/1 -> Data Type Conversion/1
  Logical Operator/1 -> Integrator/2
  ITerm_reset/1 -> Logical Operator/2
  Unit Delay/1 -> Logical Operator/1
  Constant/1 -> Unit Delay/1
  ControlHold/1 -> [HoldReq]
  [HoldReq] -> Switch2/2
  Switch2/1 -> Out/1, Unit Delay1/1
  Unit Delay1/1 -> Switch2/1
  Switch4/1 -> Product3/1
  Data Type Conversion/1 -> Control_Error/1, Switch4/3
  [HoldReq] -> Switch4/2
  Constant14/1 -> Switch4/1
  Sum1/1 -> Switch2/3
  FeedForward/1 -> Sum1/1
  D_Gain/1 -> Product4/2
  Product4/1 -> Derivative/1
  Constant1/1 -> Derivative/2
  Derivative/1 -> D_term/1, Sum/2

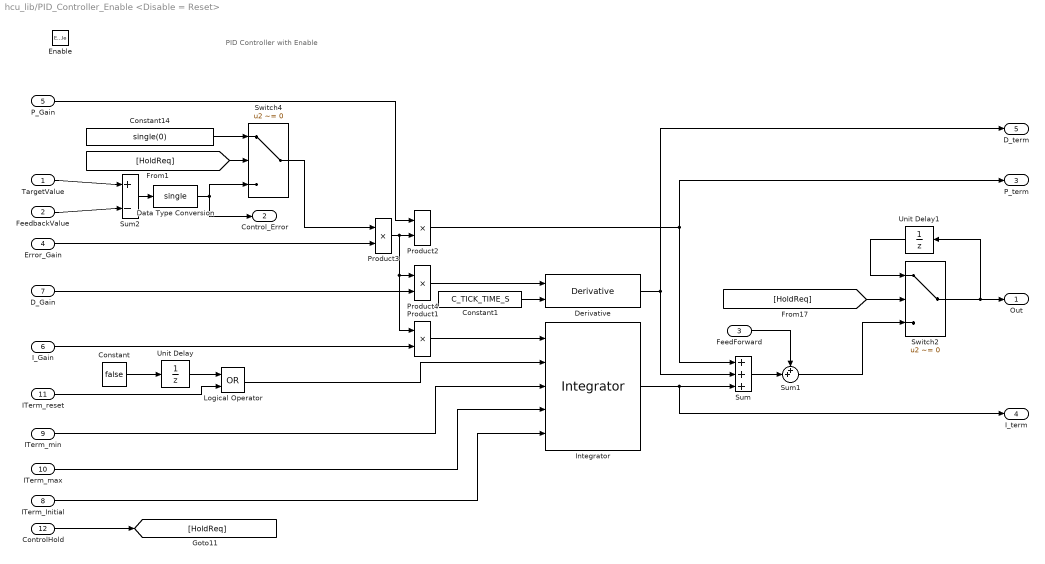
== system hcu_lib/PID_Controller_Enable <Disable = Reset> ==
  note: PID Controller with Enable
  TargetValue : Inport
  FeedbackValue : Inport  Port=2
  FeedForward : Inport  Port=3
  Error_Gain : Inport  Port=4
  P_Gain : Inport  Port=5
  I_Gain : Inport  Port=6
  D_Gain : Inport  Port=7
  ITerm_Initial : Inport  Port=8
  ITerm_min : Inport  Port=9
  ITerm_max : Inport  Port=10
  ITerm_reset : Inport  Port=11
  ControlHold : Inport  Port=12
  Enable : EnablePort  StatesWhenEnabling=reset
  Constant : Constant  Value=false  OutDataTypeStr=boolean
  Constant1 : Constant  Value=C_TICK_TIME_S  OutDataTypeStr=single
  Constant14 : Constant  Value=single(0)
  Data Type Conversion : DataTypeConversion  OutDataTypeStr=single  SaturateOnIntegerOverflow=on  RndMeth=Zero
  Derivative : hcu_lib/Derivative  SystemSampleTime=-1
  Integrator : hcu_lib/Integrator  SystemSampleTime=-1
  Logical Operator : Logic  Operator=OR  AllPortsSameDT=off  OutDataTypeStr=boolean
  Product{1..4} (4 alike) : Product  InputSameDT=on  OutDataTypeStr=Inherit: Same as first input
  Sum : Sum  Inputs=+++  SaturateOnIntegerOverflow=on  InputSameDT=on  OutDataTypeStr=Inherit: Same as first input
  Sum1 : Sum  Inputs=++|
  Sum2 : Sum  Inputs=+|-  SaturateOnIntegerOverflow=on  InputSameDT=on  OutDataTypeStr=Inherit: Same as first input
  Switch2 : Switch  Criteria=u2 ~= 0
  Switch4 : Switch  Criteria=u2 ~= 0
  Unit Delay : UnitDelay  InitialCondition=true  SampleTime=-1
  Unit Delay1 : UnitDelay  SampleTime=-1
  Out : Outport  OutputWhenDisabled=reset  InitialOutput=[0]
  Control_Error : Outport  Port=2  OutputWhenDisabled=reset  InitialOutput=[0]
  P_term : Outport  Port=3  OutputWhenDisabled=reset  InitialOutput=[0]
  I_term : Outport  Port=4  OutputWhenDisabled=reset  InitialOutput=[0]
  D_term : Outport  Port=5  OutputWhenDisabled=reset  InitialOutput=[0]
  wires:
  Derivative/1 -> Sum/2, D_term/1
  Constant1/1 -> Derivative/2
  Product4/1 -> Derivative/1
  D_Gain/1 -> Product4/2
  FeedForward/1 -> Sum1/1
  Sum1/1 -> Switch2/3
  Constant14/1 -> Switch4/1
  [HoldReq] -> Switch4/2
  Data Type Conversion/1 -> Switch4/3, Control_Error/1
  Switch4/1 -> Product3/1
  Unit Delay1/1 -> Switch2/1
  Switch2/1 -> Unit Delay1/1, Out/1
  [HoldReq] -> Switch2/2
  ControlHold/1 -> [HoldReq]
  Constant/1 -> Unit Delay/1
  Unit Delay/1 -> Logical Operator/1
  ITerm_reset/1 -> Logical Operator/2
  Logical Operator/1 -> Integrator/2
  Sum2/1 -> Data Type Conversion/1
  Product3/1 -> Product1/1, Product4/1, Product2/2
  Sum/1 -> Sum1/2
  Integrator/1 -> I_term/1, Sum/3
  Product2/1 -> Sum/1, P_term/1
  Product1/1 -> Integrator/1
  I_Gain/1 -> Product1/2
  P_Gain/1 -> Product2/1
  Error_Gain/1 -> Product3/2
  ITerm_min/1 -> Integrator/3
  ITerm_max/1 -> Integrator/4
  TargetValue/1 -> Sum2/1
  FeedbackValue/1 -> Sum2/2
  ITerm_Initial/1 -> Integrator/5

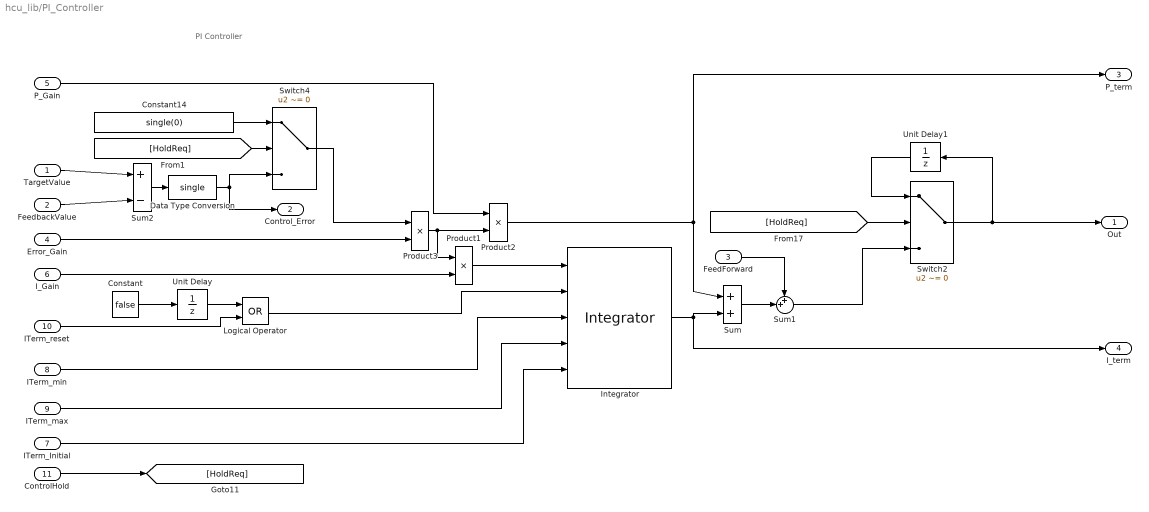
== system hcu_lib/PI_Controller ==
  note: PI Controller
  TargetValue : Inport
  FeedbackValue : Inport  Port=2
  FeedForward : Inport  Port=3
  Error_Gain : Inport  Port=4
  P_Gain : Inport  Port=5
  I_Gain : Inport  Port=6
  ITerm_Initial : Inport  Port=7
  ITerm_min : Inport  Port=8
  ITerm_max : Inport  Port=9
  ITerm_reset : Inport  Port=10
  ControlHold : Inport  Port=11
  Constant : Constant  Value=false  OutDataTypeStr=boolean
  Constant14 : Constant  Value=single(0)
  Data Type Conversion : DataTypeConversion  OutDataTypeStr=single  SaturateOnIntegerOverflow=on  RndMeth=Zero
  Integrator : hcu_lib/Integrator  SystemSampleTime=-1
  Logical Operator : Logic  Operator=OR  AllPortsSameDT=off  OutDataTypeStr=boolean
  Product1 : Product  InputSameDT=on  OutDataTypeStr=Inherit: Same as first input
  Product2 : Product  InputSameDT=on  OutDataTypeStr=Inherit: Same as first input
  Product3 : Product  InputSameDT=on  OutDataTypeStr=Inherit: Same as first input
  Sum : Sum  Inputs=+|+  SaturateOnIntegerOverflow=on  InputSameDT=on  OutDataTypeStr=Inherit: Same as first input
  Sum1 : Sum  Inputs=++|
  Sum2 : Sum  Inputs=+|-  SaturateOnIntegerOverflow=on  InputSameDT=on  OutDataTypeStr=Inherit: Same as first input
  Switch2 : Switch  Criteria=u2 ~= 0
  Switch4 : Switch  Criteria=u2 ~= 0
  Unit Delay : UnitDelay  InitialCondition=true  SampleTime=-1
  Unit Delay1 : UnitDelay  SampleTime=-1
  Out : Outport  OutputWhenDisabled=reset  InitialOutput=[0]
  Control_Error : Outport  Port=2  OutputWhenDisabled=reset  InitialOutput=[0]
  P_term : Outport  Port=3  OutputWhenDisabled=reset  InitialOutput=[0]
  I_term : Outport  Port=4  OutputWhenDisabled=reset  InitialOutput=[0]
  wires:
  FeedForward/1 -> Sum1/1
  Sum1/1 -> Switch2/3
  Constant14/1 -> Switch4/1
  [HoldReq] -> Switch4/2
  Data Type Conversion/1 -> Switch4/3, Control_Error/1
  Switch4/1 -> Product3/1
  Unit Delay1/1 -> Switch2/1
  Switch2/1 -> Unit Delay1/1, Out/1
  [HoldReq] -> Switch2/2
  ControlHold/1 -> [HoldReq]
  Constant/1 -> Unit Delay/1
  Unit Delay/1 -> Logical Operator/1
  ITerm_reset/1 -> Logical Operator/2
  Logical Operator/1 -> Integrator/2
  Sum2/1 -> Data Type Conversion/1
  Product3/1 -> Product1/1, Product2/2
  Sum/1 -> Sum1/2
  Integrator/1 -> Sum/2, I_term/1
  Product2/1 -> Sum/1, P_term/1
  Product1/1 -> Integrator/1
  I_Gain/1 -> Product1/2
  P_Gain/1 -> Product2/1
  Error_Gain/1 -> Product3/2
  ITerm_min/1 -> Integrator/3
  ITerm_max/1 -> Integrator/4
  TargetValue/1 -> Sum2/1
  FeedbackValue/1 -> Sum2/2
  ITerm_Initial/1 -> Integrator/5

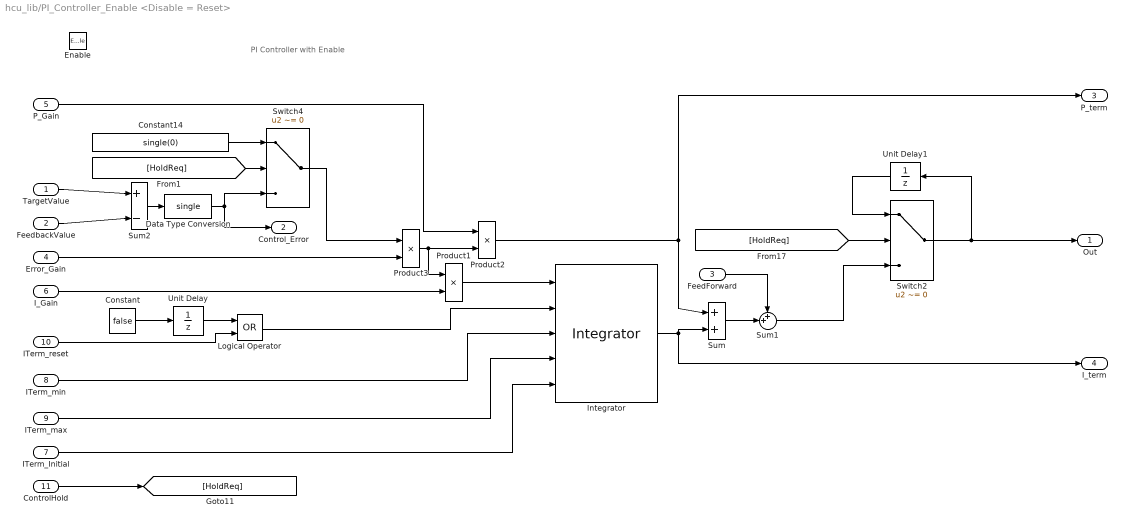
== system hcu_lib/PI_Controller_Enable <Disable = Reset> ==
  note: PI Controller with Enable
  TargetValue : Inport
  FeedbackValue : Inport  Port=2
  FeedForward : Inport  Port=3
  Error_Gain : Inport  Port=4
  P_Gain : Inport  Port=5
  I_Gain : Inport  Port=6
  ITerm_Initial : Inport  Port=7
  ITerm_min : Inport  Port=8
  ITerm_max : Inport  Port=9
  ITerm_reset : Inport  Port=10
  ControlHold : Inport  Port=11
  Enable : EnablePort  StatesWhenEnabling=reset
  Constant : Constant  Value=false  OutDataTypeStr=boolean
  Constant14 : Constant  Value=single(0)
  Data Type Conversion : DataTypeConversion  OutDataTypeStr=single  SaturateOnIntegerOverflow=on  RndMeth=Zero
  Integrator : hcu_lib/Integrator  SystemSampleTime=-1
  Logical Operator : Logic  Operator=OR  AllPortsSameDT=off  OutDataTypeStr=boolean
  Product1 : Product  InputSameDT=on  OutDataTypeStr=Inherit: Same as first input
  Product2 : Product  InputSameDT=on  OutDataTypeStr=Inherit: Same as first input
  Product3 : Product  InputSameDT=on  OutDataTypeStr=Inherit: Same as first input
  Sum : Sum  Inputs=+|+  SaturateOnIntegerOverflow=on  InputSameDT=on  OutDataTypeStr=Inherit: Same as first input
  Sum1 : Sum  Inputs=++|
  Sum2 : Sum  Inputs=+|-  SaturateOnIntegerOverflow=on  InputSameDT=on  OutDataTypeStr=Inherit: Same as first input
  Switch2 : Switch  Criteria=u2 ~= 0
  Switch4 : Switch  Criteria=u2 ~= 0
  Unit Delay : UnitDelay  InitialCondition=true  SampleTime=-1
  Unit Delay1 : UnitDelay  SampleTime=-1
  Out : Outport  OutputWhenDisabled=reset  InitialOutput=[0]
  Control_Error : Outport  Port=2  OutputWhenDisabled=reset  InitialOutput=[0]
  P_term : Outport  Port=3  OutputWhenDisabled=reset  InitialOutput=[0]
  I_term : Outport  Port=4  OutputWhenDisabled=reset  InitialOutput=[0]
  wires:
  FeedbackValue/1 -> Sum2/2
  TargetValue/1 -> Sum2/1
  ITerm_max/1 -> Integrator/4
  ITerm_min/1 -> Integrator/3
  Error_Gain/1 -> Product3/2
  P_Gain/1 -> Product2/1
  I_Gain/1 -> Product1/2
  Product1/1 -> Integrator/1
  Product2/1 -> P_term/1, Sum/1
  Integrator/1 -> I_term/1, Sum/2
  Sum/1 -> Sum1/2
  Product3/1 -> Product2/2, Product1/1
  Sum2/1 -> Data Type Conversion/1
  Logical Operator/1 -> Integrator/2
  ITerm_reset/1 -> Logical Operator/2
  Unit Delay/1 -> Logical Operator/1
  Constant/1 -> Unit Delay/1
  ControlHold/1 -> [HoldReq]
  [HoldReq] -> Switch2/2
  Switch2/1 -> Out/1, Unit Delay1/1
  Unit Delay1/1 -> Switch2/1
  Switch4/1 -> Product3/1
  Data Type Conversion/1 -> Control_Error/1, Switch4/3
  [HoldReq] -> Switch4/2
  Constant14/1 -> Switch4/1
  Sum1/1 -> Switch2/3
  FeedForward/1 -> Sum1/1
  ITerm_Initial/1 -> Integrator/5
